simulink model "Saturation_Mask"  (R2021a)
settings: Solver=VariableStepAuto  StartTime=0.0  StopTime=10.0  RelTol=1e-3
settings Model: Creator=lenovo  LastModifiedBy=lenovo

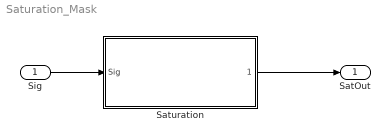
== system Saturation_Mask ==
  Sig : Inport
  Saturation : Subsystem  mask{UL=0, LL=0}
      mask prompts: UL "Upper Limit"; LL "Lower Limit"
      mask DialogControl DescGroupVar Prompt: Saturation
      mask DialogControl DescTextVar Prompt: This Block for saturation of input signal
  SatOut : Outport
  wires:
  Sig/1 -> Saturation/1(Sig)
  Saturation/1(1) -> SatOut/1

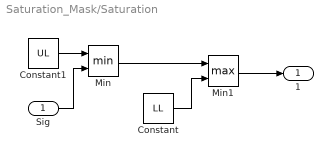
== system Saturation_Mask/Saturation ==
  Sig : Inport
  Constant : Constant  Value=LL
  Constant1 : Constant  Value=UL
  Min : MinMax  Inputs=2
  Min1 : MinMax  Function=max  Inputs=2
  1 : Outport
  wires:
  Min/1 -> Min1/1
  Sig/1 -> Min/2
  Constant/1 -> Min1/2
  Min1/1 -> 1/1
  Constant1/1 -> Min/1
